simulink model "tests_airgap2pos"  (R2022b)
settings: Solver=VariableStepAuto  StartTime=0.0  StopTime=10.0  RelTol=1e-3
values from neighbouring files (symbols this model uses):
  airgap1 = -abs(airgap1-airgap1(1))+22.5    [graficasLevitacion.m]
  airgap2 = -abs(airgap2-airgap2(1))+22.5    [graficasLevitacion.m]
  airgap3 = -abs(airgap3-airgap3(1))+22.5    [graficasLevitacion.m]
  airgap4 = -abs(airgap4-airgap4(1))+22.5    [graficasLevitacion.m]
  airgap5 = 100-airgap5    [graficasLevitacion.m]
  airgap6 = 100-airgap6    [graficasLevitacion.m]
  airgap7 = 100-airgap7    [graficasLevitacion.m]
  airgap8 = 100-airgap8    [graficasLevitacion.m]
settings Model: Creator=ramuj  LastModifiedBy=ramuj

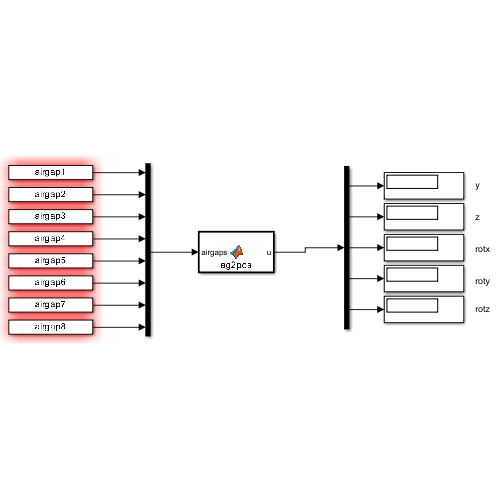
[thumbnail: Simulink's stored preview of the top-level diagram]
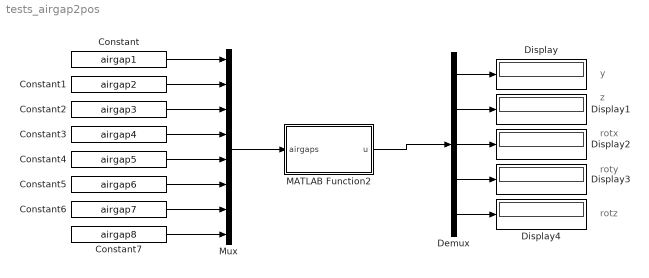
== system tests_airgap2pos ==
  note: y
  note: z
  note: rotx
  note: roty
  note: rotz
  Constant : Constant  Value=airgap1
  Constant1 : Constant  Value=airgap2
  Constant2 : Constant  Value=airgap3
  Constant3 : Constant  Value=airgap4
  Constant4 : Constant  Value=airgap5
  Constant5 : Constant  Value=airgap6
  Constant6 : Constant  Value=airgap7
  Constant7 : Constant  Value=airgap8
  Demux : Demux  Outputs=5
  Display{,1..4} (5 alike) : Display
  MATLAB Function2 : MATLAB Function  TreatAsAtomicUnit=on
  Mux : Mux  Inputs=8
  wires:
  Mux/1 -> MATLAB Function2/1(airgaps)
  Constant/1 -> Mux/1
  Constant1/1 -> Mux/2
  Constant2/1 -> Mux/3
  Constant3/1 -> Mux/4
  Constant4/1 -> Mux/5
  Constant5/1 -> Mux/6
  Constant6/1 -> Mux/7
  Constant7/1 -> Mux/8
  MATLAB Function2/1(u) -> Demux/1
  Demux/1 -> Display/1
  Demux/2 -> Display1/1
  Demux/3 -> Display2/1
  Demux/4 -> Display3/1
  Demux/5 -> Display4/1

== matlab function tests_airgap2pos/MATLAB Function2 ==
  data: airgaps input; u output
function u = ag2pos(airgaps)

% CONSTANTES
x_sragy = 0.7681;
y_sragy = 0.0951;
z_sragy = 0.07922;
x_sragz = 0.76785;
y_sragz = 0.22269;
z_sragz = -0.09493;
z_infr = 0.6328;
grosorz = 0.015;
grosory = 0.005;

coder.varsize('rotx_aux');
coder.varsize('roty_aux');
coder.varsize('rotz_aux');
coder.varsize('y_aux');
coder.varsize('z_aux');

rotx_aux=zeros(2,1);
roty_aux=zeros(2,1);
rotz_aux=zeros(2,1);
y_aux=zeros(4,1);
z_aux=zeros(4,1);

% ROTACIONES
rotx_aux(1) = asin((airgaps(2) - airgaps(1))/(2*y_sragz));
rotx_aux(2) = asin((airgaps(4) - airgaps(3))/(2*y_sragz));

roty_aux(1) = asin((airgaps(1) - airgaps(3))/(2*x_sragz));
roty_aux(2) = asin((airgaps(2) - airgaps(4))/(2*x_sragz));

rotz_aux(1) = asin((airgaps(5) - airgaps(7))/(2*x_sragy));
rotz_aux(2) = asin((airgaps(8) - airgaps(6))/(2*x_sragy));

rotx = mean(rotx_aux);
roty = mean(roty_aux);
rotz = mean(rotz_aux);

% DISTANCIAS
y_aux(1) = + airgaps(5) - y_sragy * cos(rotz) - x_sragy * sin(rotz) + z_sragy * sin(rotx) + grosory;
y_aux(2) = - airgaps(6) + y_sragy * cos(rotz) - x_sragy * sin(rotz) + z_sragy * sin(rotx) - grosory;
y_aux(3) = + airgaps(7) - y_sragy * cos(rotz) + x_sragy * sin(rotz) + z_sragy * sin(rotx) + grosory;
y_aux(4) = - airgaps(8) + y_sragy * cos(rotz) + x_sragy * sin(rotz) + z_sragy * sin(rotx) - grosory;

z_aux(1) = z_infr - airgaps(1) - z_sragz * cos(roty) + x_sragz * sin(roty) - y_sragz * sin(rotx);
z_aux(2) = z_infr - airgaps(2) - z_sragz * cos(roty) + x_sragz * sin(roty) + y_sragz * sin(rotx);
z_aux(3) = z_infr - airgaps(3) - z_sragz * cos(roty) - x_sragz * sin(roty) - y_sragz * sin(rotx);
z_aux(4) = z_infr - airgaps(4) - z_sragz * cos(roty) - x_sragz * sin(roty) + y_sragz * sin(rotx);

y = mean(y_aux);
z = mean(z_aux);
u =[y, z, rotx, roty, rotz]';
